simulink model "SeatControlSCS"  (R2025a)
settings: Solver=ode4  StopTime=30  FixedStep=0.01
libraries: simulink x2
settings Model: Creator=amith  LastModifiedBy=amith

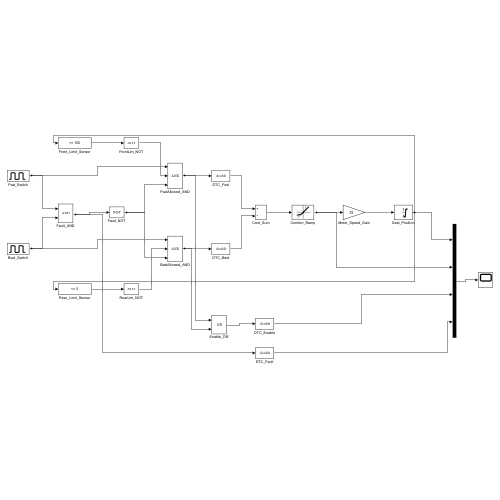
[thumbnail: Simulink's stored preview of the top-level diagram]
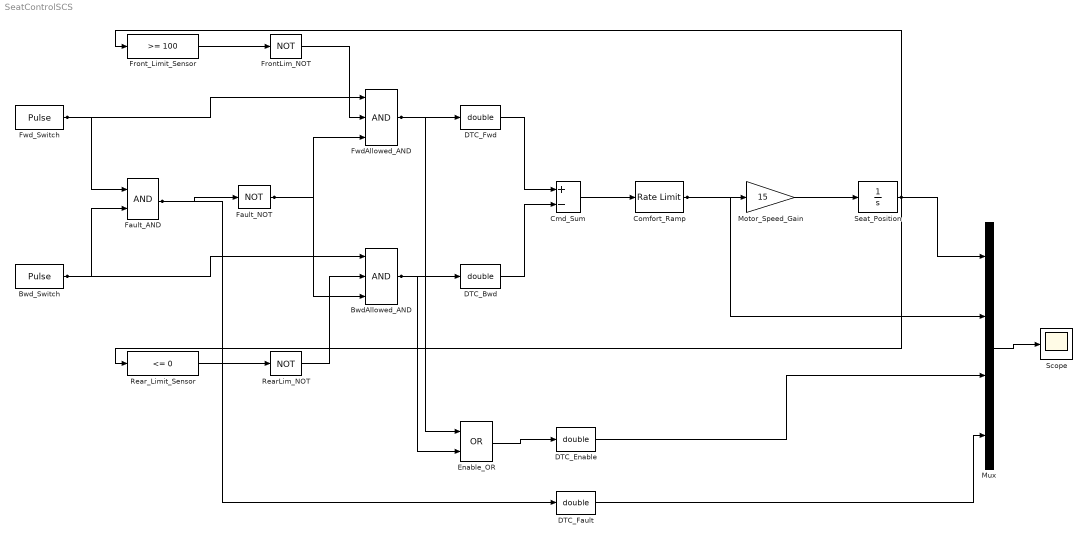
== system SeatControlSCS ==
  BwdAllowed_AND : Logic  Inputs=3  AllPortsSameDT=off  OutDataTypeStr=boolean
  Bwd_Switch : DiscretePulseGenerator  PulseType=Time based  Period=30  PulseWidth=20  PhaseDelay=15
  Cmd_Sum : Sum  Inputs=+-
  Comfort_Ramp : RateLimiter  RisingSlewLimit=2  FallingSlewLimit=-2  SampleTimeMode=inherited
  DTC_Bwd : DataTypeConversion  OutDataTypeStr=double  SaturateOnIntegerOverflow=off  RndMeth=Floor
  DTC_Enable : DataTypeConversion  OutDataTypeStr=double  SaturateOnIntegerOverflow=off  RndMeth=Floor
  DTC_Fault : DataTypeConversion  OutDataTypeStr=double  SaturateOnIntegerOverflow=off  RndMeth=Floor
  DTC_Fwd : DataTypeConversion  OutDataTypeStr=double  SaturateOnIntegerOverflow=off  RndMeth=Floor
  Enable_OR : Logic  Operator=OR  AllPortsSameDT=off  OutDataTypeStr=boolean
  Fault_AND : Logic  AllPortsSameDT=off  OutDataTypeStr=boolean
  Fault_NOT : Logic  Operator=NOT  AllPortsSameDT=off  OutDataTypeStr=boolean
  FrontLim_NOT : Logic  Operator=NOT  AllPortsSameDT=off  OutDataTypeStr=boolean
  Front_Limit_Sensor : simulink/Logic and Bit Operations/Compare To Constant  relop=>=  const=100  OutDataTypeStr=boolean
  FwdAllowed_AND : Logic  Inputs=3  AllPortsSameDT=off  OutDataTypeStr=boolean
  Fwd_Switch : DiscretePulseGenerator  PulseType=Time based  Period=30  PulseWidth=30
  Motor_Speed_Gain : Gain  Gain=15
  Mux : Mux
  RearLim_NOT : Logic  Operator=NOT  AllPortsSameDT=off  OutDataTypeStr=boolean
  Rear_Limit_Sensor : simulink/Logic and Bit Operations/Compare To Constant  relop=<=  const=0  OutDataTypeStr=boolean
  Scope : Scope
  Seat_Position : Integrator  LimitOutput=on  UpperSaturationLimit=100  LowerSaturationLimit=0
  wires:
  Fwd_Switch/1 -> Fault_AND/1, FwdAllowed_AND/1
  Bwd_Switch/1 -> Fault_AND/2, BwdAllowed_AND/1
  Fault_AND/1 -> Fault_NOT/1, DTC_Fault/1
  Front_Limit_Sensor/1 -> FrontLim_NOT/1
  Rear_Limit_Sensor/1 -> RearLim_NOT/1
  FrontLim_NOT/1 -> FwdAllowed_AND/2
  Fault_NOT/1 -> FwdAllowed_AND/3, BwdAllowed_AND/3
  RearLim_NOT/1 -> BwdAllowed_AND/2
  FwdAllowed_AND/1 -> Enable_OR/1, DTC_Fwd/1
  BwdAllowed_AND/1 -> Enable_OR/2, DTC_Bwd/1
  DTC_Fwd/1 -> Cmd_Sum/1
  DTC_Bwd/1 -> Cmd_Sum/2
  Cmd_Sum/1 -> Comfort_Ramp/1
  Comfort_Ramp/1 -> Motor_Speed_Gain/1, Mux/2
  Motor_Speed_Gain/1 -> Seat_Position/1
  Seat_Position/1 -> Front_Limit_Sensor/1, Rear_Limit_Sensor/1, Mux/1
  Enable_OR/1 -> DTC_Enable/1
  DTC_Enable/1 -> Mux/3
  DTC_Fault/1 -> Mux/4
  Mux/1 -> Scope/1
